simulink model "ShubhamGupta_180749_Lab2"  (R2020b)
settings: Solver=ode2  StartTime=0.0  StopTime=50  FixedStep=0.1  RelTol=1e-3  EnableMultiTasking=on
undefined symbols (not defined in the file or in its folder): B, Tic
settings Model: Creator=HP  LastModifiedBy=subhamgupta
settings DataIOCC: ReturnWorkspaceOutputs=off
settings OptimizationCC: LifeSpan=inf
settings DebuggingCC: SFUnexpectedBacktrackingDiag=warning  SFNoUnconditionalDefaultTransitionDiag=warning  ArithmeticOperatorsInVariantConditions=warning
settings SFSimCC: SimUseLocalCustomCode=off  CustomCodeUndefinedFunction=UseInterfaceOnly
settings RTWCC: RTWUseLocalCustomCode=off
settings CodeAppCC: StateflowObjectComments=on
settings GRTTargetCC: TargetLangStandard=C89/C90 (ANSI)
settings ConfigComp: CovMetricSettings=dw  CovSaveCumulativeToWorkspaceVar=on  CovSaveSingleToWorkspaceVar=on  CovExternalEMLEnable=off

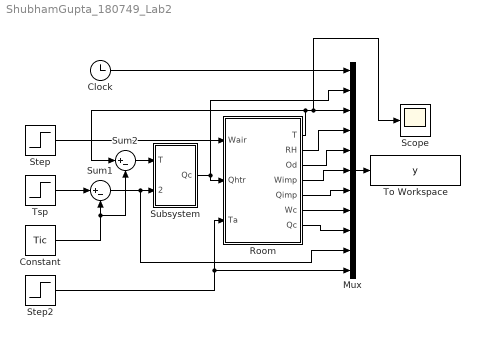
== system ShubhamGupta_180749_Lab2 ==
  Clock : Clock
  Constant : Constant  Value=Tic
  Mux : Mux  Inputs=11
  Room : Subsystem  mask{Qic=50, Wic=0, Tic=25, RHic=30}
      mask prompts: Qic "Qhtr Initial Condition"; Wic "Wair Initial Condition"; Tic "T Initial Condition"; RHic "RH Initial Condition"
  Scope : Scope
  Step : Step  Time=0  After=0  SampleTime=0
  Step2 : Step  Time=0  After=0  SampleTime=0
  Subsystem : Subsystem  mask{Kc=6.0384, Ti=18.9142, Td=0, k=Reverse}
      mask prompts: Kc "Controller Gain"; Ti "Integral Time"; Td "Derivative Time"; k "Controller Action"
      mask TypeOptions k: Reverse  | Direct
  Sum1 : Sum  Inputs=|+-
  Sum2 : Sum  Inputs=|+-
  To Workspace : ToWorkspace  VariableName=y  SampleTime=-1
  Tsp : Step  Time=0  Before=25  After=26  SampleTime=0
  wires:
  Clock/1 -> Mux/1
  Room/1(T) -> Sum2/1, Scope/1, Mux/3
  Room/2(RH) -> Mux/4
  Room/3(Od) -> Mux/5
  Room/4(Wimp) -> Mux/6
  Room/5(Qimp) -> Mux/7
  Room/6(Wc) -> Mux/8
  Room/7(Qc) -> Mux/9
  Mux/1 -> To Workspace/1
  Subsystem/1(Qc) -> Mux/2, Room/2(Qhtr)
  Step/1 -> Room/1(Wair)
  Step2/1 -> Room/3(Ta), Mux/11
  Tsp/1 -> Sum1/1
  Constant/1 -> Sum2/2, Sum1/2
  Sum1/1 -> Mux/10, Subsystem/2(Tsp)
  Sum2/1 -> Subsystem/1(T)

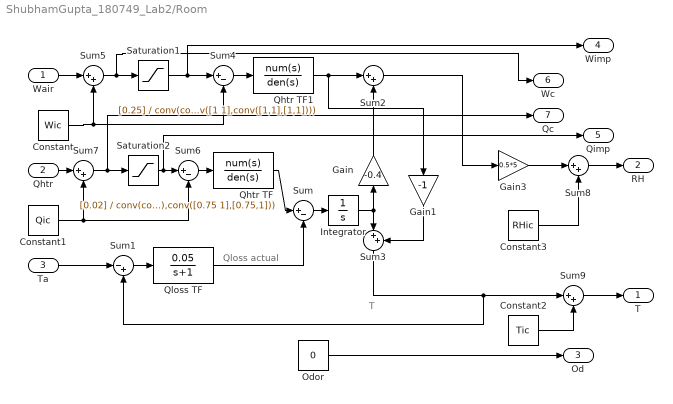
== system ShubhamGupta_180749_Lab2/Room ==
  note: Qloss actual
  note: T
  Wair : Inport
  Qhtr : Inport  Port=2
  Ta : Inport  Port=3
  Constant : Constant  Value=Wic
  Constant1 : Constant  Value=Qic
  Constant2 : Constant  Value=Tic
  Constant3 : Constant  Value=RHic
  Gain : Gain  Gain=-0.4
  Gain1 : Gain  Gain=-1
  Gain3 : Gain  Gain=0.5*5
  Integrator : Integrator
  Odor : Constant  Value=0
  Qhtr TF : TransferFcn  Numerator=[0.02]  Denominator=conv(conv(conv([0.75 1],[0.75,1]),[0.75 1]),conv([0.75 1],[0.75,1]))
  Qhtr TF1 : TransferFcn  Numerator=[0.25]  Denominator=conv(conv([1 1],conv([1,1],[1,1])),conv([1 1],conv([1,1],[1,1])))
  Qloss TF : TransferFcn  Numerator=[0.05]  Denominator=[1 1]
  Saturation1 : Saturate  UpperLimit=100  LowerLimit=0
  Saturation2 : Saturate  UpperLimit=100  LowerLimit=0
  Sum : Sum  Inputs=|+-
  Sum1 : Sum  Inputs=|-+
  Sum{2..3,5,7..9} (6 alike) : Sum  Inputs=|++
  Sum4 : Sum  Inputs=|+-
  Sum6 : Sum  Inputs=|+-
  T : Outport
  RH : Outport  Port=2
  Od : Outport  Port=3
  Wimp : Outport  Port=4
  Qimp : Outport  Port=5
  Wc : Outport  Port=6
  Qc : Outport  Port=7
  wires:
  Qhtr TF/1 -> Sum/1
  Gain/1 -> Sum2/2
  Qloss TF/1 -> Sum/2
  Integrator/1 -> Gain/1, Sum3/1
  Gain1/1 -> Sum3/2
  Odor/1 -> Od/1
  Ta/1 -> Sum1/1
  Sum/1 -> Integrator/1
  Sum1/1 -> Qloss TF/1
  Qhtr TF1/1 -> Gain1/1, Sum2/1
  Sum3/1 -> Sum1/2, Sum9/1
  Sum2/1 -> Gain3/1
  Saturation1/1 -> Wimp/1, Sum4/1
  Sum4/1 -> Qhtr TF1/1
  Wair/1 -> Sum5/1
  Sum5/1 -> Wc/1, Saturation1/1
  Saturation2/1 -> Qimp/1, Sum6/1
  Sum6/1 -> Qhtr TF/1
  Qhtr/1 -> Sum7/1
  Sum7/1 -> Qc/1, Saturation2/1
  Gain3/1 -> Sum8/1
  Sum8/1 -> RH/1
  Sum9/1 -> T/1
  Constant/1 -> Sum4/2, Sum5/2
  Constant1/1 -> Sum6/2, Sum7/2
  Constant3/1 -> Sum8/2
  Constant2/1 -> Sum9/2

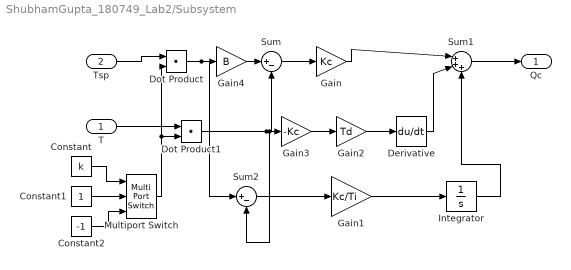
== system ShubhamGupta_180749_Lab2/Subsystem ==
  T : Inport
  Tsp : Inport  Port=2
  Constant : Constant  Value=k
  Constant1 : Constant
  Constant2 : Constant  Value=-1
  Derivative : Derivative
  Dot Product : DotProduct  InputSameDT=on  OutDataTypeStr=Inherit: Inherit via internal rule
  Dot Product1 : DotProduct  InputSameDT=on  OutDataTypeStr=Inherit: Inherit via internal rule
  Gain : Gain  Gain=Kc
  Gain1 : Gain  Gain=Kc/Ti
  Gain2 : Gain  Gain=Td
  Gain3 : Gain  Gain=-Kc
  Gain4 : Gain  Gain=B
  Integrator : Integrator
  Multiport Switch : MultiPortSwitch  Inputs=2
  Sum : Sum  Inputs=|+-
  Sum1 : Sum  Inputs=|+++
  Sum2 : Sum  Inputs=|+-
  Qc : Outport
  wires:
  Sum1/1 -> Qc/1
  Sum/1 -> Gain/1
  Derivative/1 -> Sum1/2
  Gain3/1 -> Gain2/1
  Gain/1 -> Sum1/1
  Gain2/1 -> Derivative/1
  Constant/1 -> Multiport Switch/1
  Constant1/1 -> Multiport Switch/2
  Constant2/1 -> Multiport Switch/3
  Tsp/1 -> Dot Product/1
  Multiport Switch/1 -> Dot Product1/2, Dot Product/2
  T/1 -> Dot Product1/1
  Dot Product1/1 -> Sum2/2, Sum/2, Gain3/1
  Dot Product/1 -> Sum2/1, Gain4/1
  Gain4/1 -> Sum/1
  Gain1/1 -> Integrator/1
  Sum2/1 -> Gain1/1
  Integrator/1 -> Sum1/3
